simulink model "basebot_drive"  (R2025a)
settings: Solver=ode45  StartTime=0.0  StopTime=1.5  RelTol=1e-3
InitFcn:
  | if exist('piDesign.mat','file'), load('piDesign.mat'); end; gear=9.6; wrad=0.0315; B=0.15; limit_9V=9; Ts=0.001;
values from neighbouring files (symbols this model uses):
  den = [4.84323072847e-08 4.8661333765e-05 8.000321026e-05]    [piDesign.mat]    (also in transferFunction.m = conv([L R], [J D]) + [0 0 K^2])
  Kp = 0.2    [piDesign.m]    (also in piDesign.mat)
  num = 0.00868283239801    [piDesign.mat]    (also in transferFunction.m = K)
settings Model: Creator=leon3  LastModifiedBy=leon3

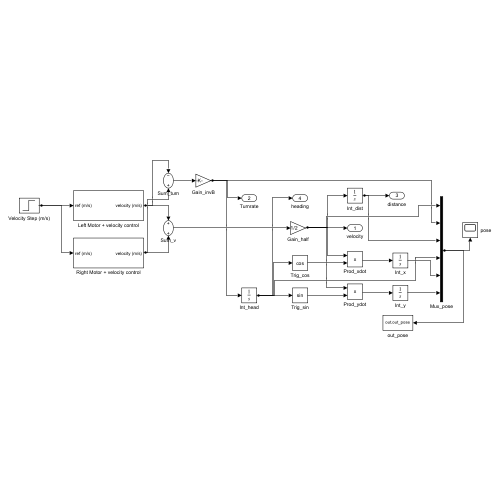
[thumbnail: Simulink's stored preview of the top-level diagram]
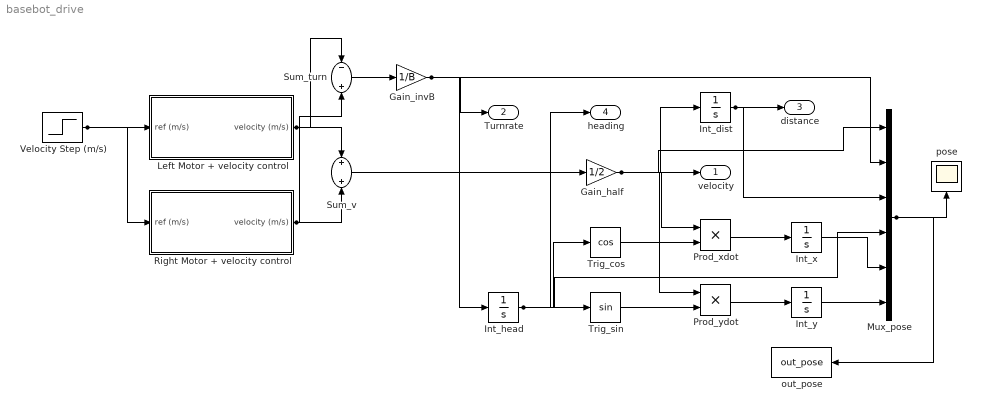
== system basebot_drive ==
  Gain_half : Gain  Gain=1/2
  Gain_invB : Gain  Gain=1/B
  Int_dist : Integrator
  Int_head : Integrator
  Int_x : Integrator
  Int_y : Integrator
  Left Motor + velocity control : Subsystem
  Mux_pose : Mux  Inputs=6
  Prod_xdot : Product  Inputs=**
  Prod_ydot : Product  Inputs=**
  Right Motor + velocity control : Subsystem
  Sum_turn : Sum  Inputs=-+
  Sum_v : Sum
  Trig_cos : Trigonometry  Operator=cos
  Trig_sin : Trigonometry
  Velocity Step (m/s) : Step  Time=0.1  After=0.4  SampleTime=0
  out_pose : ToWorkspace  VariableName=out_pose  SaveFormat=Timeseries  SampleTime=-1
  pose : Scope
  velocity : Outport
  Turnrate : Outport  Port=2
  distance : Outport  Port=3
  heading : Outport  Port=4
  wires:
  Gain_half/1 -> Int_dist/1, velocity/1, Prod_ydot/1, Prod_xdot/1, Mux_pose/1
  Velocity Step (m/s)/1 -> Left Motor + velocity control/1(ref (m/s)), Right Motor + velocity control/1(ref (m/s))
  Sum_v/1 -> Gain_half/1
  Left Motor + velocity control/1(velocity (m/s)) -> Sum_turn/1, Sum_v/1
  Right Motor + velocity control/1(velocity (m/s)) -> Sum_v/2, Sum_turn/2
  Gain_invB/1 -> Mux_pose/2, Int_head/1, Turnrate/1
  Sum_turn/1 -> Gain_invB/1
  Int_head/1 -> Trig_sin/1, heading/1, Trig_cos/1, Mux_pose/4
  Prod_xdot/1 -> Int_x/1
  Trig_cos/1 -> Prod_xdot/2
  Trig_sin/1 -> Prod_ydot/2
  Int_dist/1 -> Mux_pose/3, distance/1
  Prod_ydot/1 -> Int_y/1
  Int_x/1 -> Mux_pose/5
  Int_y/1 -> Mux_pose/6
  Mux_pose/1 -> pose/1, out_pose/1

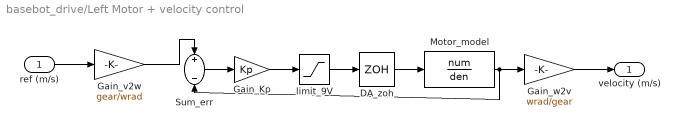
== system basebot_drive/Left Motor + velocity control ==
  ref (m/s) : Inport
  DA_zoh : ZeroOrderHold  SampleTime=0.001
  Gain_Kp : Gain  Gain=Kp
  Gain_v2w : Gain  Gain=gear/wrad
  Gain_w2v : Gain  Gain=wrad/gear
  Motor_model : TransferFcn  Numerator=num  Denominator=den
  Sum_err : Sum  Inputs=+-
  limit_9V : Saturate  UpperLimit=9  LowerLimit=-9
  velocity (m/s) : Outport
  wires:
  ref (m/s)/1 -> Gain_v2w/1
  Gain_v2w/1 -> Sum_err/1
  Sum_err/1 -> Gain_Kp/1
  Gain_Kp/1 -> limit_9V/1
  limit_9V/1 -> DA_zoh/1
  DA_zoh/1 -> Motor_model/1
  Motor_model/1 -> Gain_w2v/1, Sum_err/2
  Gain_w2v/1 -> velocity (m/s)/1

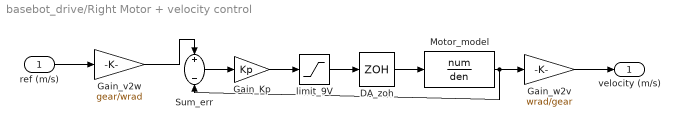
== system basebot_drive/Right Motor + velocity control ==
  ref (m/s) : Inport
  DA_zoh : ZeroOrderHold  SampleTime=0.001
  Gain_Kp : Gain  Gain=Kp
  Gain_v2w : Gain  Gain=gear/wrad
  Gain_w2v : Gain  Gain=wrad/gear
  Motor_model : TransferFcn  Numerator=num  Denominator=den
  Sum_err : Sum  Inputs=+-
  limit_9V : Saturate  UpperLimit=9  LowerLimit=-9
  velocity (m/s) : Outport
  wires:
  ref (m/s)/1 -> Gain_v2w/1
  Gain_v2w/1 -> Sum_err/1
  Sum_err/1 -> Gain_Kp/1
  Gain_Kp/1 -> limit_9V/1
  limit_9V/1 -> DA_zoh/1
  DA_zoh/1 -> Motor_model/1
  Motor_model/1 -> Gain_w2v/1, Sum_err/2
  Gain_w2v/1 -> velocity (m/s)/1
